simulink model "UseCase_v3"  (R2024b)
settings: Solver=ode1  StartTime=0.0  StopTime=365*24  FixedStep=0.05  RelTol=1e-3
libraries: filter_lib x5, buffer_lib x3, storage_lib x2, transport_lib x1
settings Model: SimulationMode=accelerator  Creator=marcv  LastModifiedBy=marcv
settings RTWCC: GPUComputeCapability=3.5

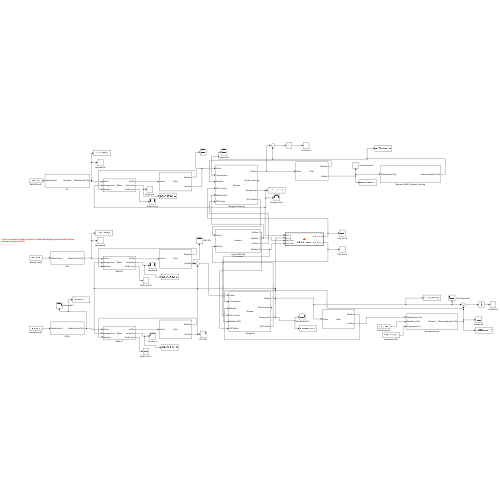
[thumbnail: Simulink's stored preview of the top-level diagram]
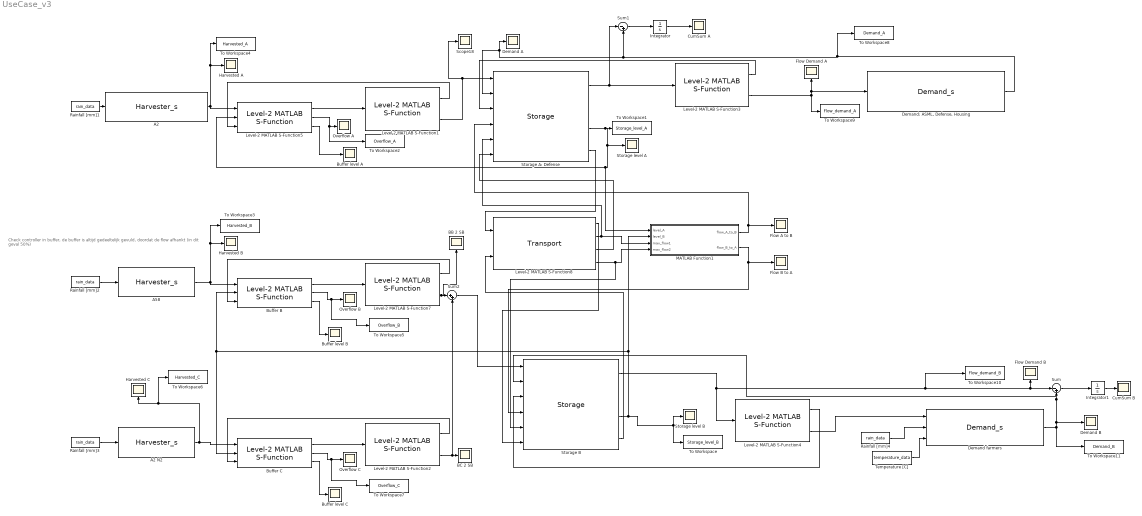
== system UseCase_v3 ==
  note: Check controller in buffer, de buffer is altijd gedeeltelijk gevuld, doordat de flow afhankt (in dit geval 50%)
  A2 : M-S-Function  FunctionName=Harvester_s  Parameters=Type_harvester, inflow_groundwater, Area  mask{Type_harvester=Dependant on ground water (tunnel), inflow_groundwater=91, Area=64000}
      mask prompts: Type_harvester "Type of harvester:"; inflow_groundwater "Inflow groundwater [m^3/h]:"; Area "Area [m^2]:"
      mask DialogControl DescGroupVar Prompt: Harvester
      mask DialogControl DescTextVar Prompt: Text
      mask Display:
      | disp('Harvester')
      | port_label('input', 1, 'Rainfall [mm]');
      | port_label('output', 1, 'Waterflow [m^3/h]');
  A2 N2 : M-S-Function  FunctionName=Harvester_s  Parameters=Type_harvester, inflow_groundwater, Area  mask{Type_harvester=Independant on ground water (resevoir, road ect.), inflow_groundwater=20, Area=21e4}
      mask prompts: Type_harvester "Type of harvester:"; inflow_groundwater "Inflow groundwater [m^3/h]:"; Area "Area [m^2]:"
      mask DialogControl DescGroupVar Prompt: Harvester
      mask DialogControl DescTextVar Prompt: Text
      mask Display:
      | port_label('input', 1, 'Rainfall [mm]');
      | port_label('output', 1, 'Waterflow [m^3/h]');
  A58 : M-S-Function  FunctionName=Harvester_s  Parameters=Type_harvester, inflow_groundwater, Area  mask{Type_harvester=Independant on ground water (resevoir, road ect.), inflow_groundwater=20, Area=13.5e4}
      mask prompts: Type_harvester "Type of harvester:"; inflow_groundwater "Inflow groundwater [m^3/h]:"; Area "Area [m^2]:"
      mask DialogControl DescGroupVar Prompt: Harvester
      mask DialogControl DescTextVar Prompt: Text
      mask Display:
      | port_label('input', 1, 'Rainfall [mm]');
      | port_label('output', 1, 'Waterflow [m^3/h]');
  BB 2 SB : Scope
  BC 2 SB : Scope
  Buffer B : buffer_lib/Level-2 MATLAB S-Function  Parameter1=7e3
  Buffer C : buffer_lib/Level-2 MATLAB S-Function  Parameter1=1e4
  Buffer level A : Scope
  Buffer level B : Scope
  Buffer level C : Scope
  CumSum A : Scope
  CumSum B : Scope
  Demand A : Scope
  Demand B : Scope
  Demand farmers : M-S-Function  FunctionName=Demand_s  Parameters=Type_demand, Constant_demand, Crop_type, Area  mask{Type_demand=Agriculture, Constant_demand=0, Crop_type=Potato, Area=3e5}
      mask prompts: Type_demand "Type of demand:"; Constant_demand "Demand [m^3/y]:"; Crop_type "Crop type:"; Area "Area [m^2]:"
      mask DialogControl DescGroupVar Prompt: Demand
      mask DialogControl DescTextVar Prompt: Demand text
      mask Display:
      | disp('Demand')
      | 
      | port_label('input', 1, 'Waterflow [m^3/h]');
      | if get_param(gcb, 'Type_demand') == "Agriculture"
      |     port_label('input', 2, 'Rainfall [m^3/h]');
      |     port_label('input', 3, 'Temperature [C]');
      | end
      | 
      | port_label('output', 1, 'Water demand [m^3/h]');
  "Demand: ASML, Defense, Housing" : M-S-Function  FunctionName=Demand_s  Parameters=Type_demand, Constant_demand, Crop_type, Area  mask{Type_demand=Constant demand, Constant_demand=8e5, Crop_type=Spinach, Area=3500000}
      mask prompts: Type_demand "Type of demand:"; Constant_demand "Demand [m^3/y]:"; Crop_type "Crop type:"; Area "Area [m^2]:"
      mask DialogControl DescGroupVar Prompt: Demand
      mask DialogControl DescTextVar Prompt: Demand text
      mask Display:
      | port_label('input', 1, 'Waterflow [m^3/h]');
      | if get_param(gcb, 'Type_demand') == "Agriculture"
      |     port_label('input', 2, 'Rainfall [m^3/h]');
      | end
      | 
      | port_label('output', 1, 'Water demand [m^3/h]');
  Flow A to B : Scope
  Flow B to A : Scope
  Flow Demand A : Scope
  Flow Demand B : Scope
  Harvested A : Scope
  Harvested B : Scope
  Harvested C : Scope
  Integrator : Integrator
  Integrator1 : Integrator
  Level-2 MATLAB S-Function1 : filter_lib/Level-2 MATLAB S-Function  filteroption=Custom filter  Parameter4=Cyclone-sand-UV [90 m3/h]  Parameter1=200  Parameter2=1
  Level-2 MATLAB S-Function2 : filter_lib/Level-2 MATLAB S-Function  filteroption=Custom filter  Parameter4=Cyclone-sand-UV [90 m3/h]  Parameter1=100  Parameter2=1
  Level-2 MATLAB S-Function3 : filter_lib/Level-2 MATLAB S-Function  filteroption=Custom filter  Parameter4=Cyclone-sand-UV [90 m3/h]  Parameter1=100  Parameter2=1
  Level-2 MATLAB S-Function4 : filter_lib/Level-2 MATLAB S-Function  filteroption=Custom filter  Parameter4=Cyclone-sand-UV [90 m3/h]  Parameter1=400  Parameter2=1
  Level-2 MATLAB S-Function5 : buffer_lib/Level-2 MATLAB S-Function  Parameter1=1e4
  Level-2 MATLAB S-Function7 : filter_lib/Level-2 MATLAB S-Function  filteroption=Custom filter  Parameter4=Cyclone-sand-UV [90 m3/h]  Parameter1=100  Parameter2=1
  Level-2 MATLAB S-Function8 : transport_lib/Transport  max_flow_result1=195.5517  max_flow_result2=188.5717  flowDirec=Bidirectional  setupopt=Transport only  Transporttype=Custom  Dist=20000  elevation=1  width=1  depth=3  diameter=0.3  dP=3  customflow=200  filteroption=Common filter  Fflowmax=3000  dPfilter=1  selectedfilter=Reverse Osmosis [27 m3/h (PureAqua TW-173K-4680)]  filterparallel=2
  MATLAB Function1 : MATLAB Function  TreatAsAtomicUnit=on
  Overflow A : Scope
  Overflow B : Scope
  Overflow C : Scope
  Rainfall [mm]{1..4} (4 alike) : FromWorkspace  VariableName=rain_data  OutDataTypeStr=double  SampleTime=1
  Scope18 : Scope
  Storage A: Defense : storage_lib/Storage  Parameter1=22.5e4  Parameter2=0.6  Parameter3=1 interconnection
  Storage B : storage_lib/Storage  Parameter1=5e4  Parameter2=0.6  Parameter3=1 interconnection
  Storage level A : Scope
  Storage level B : Scope
  Sum : Sum  Inputs=|-+
  Sum1 : Sum  Inputs=|-+
  Sum2 : Sum  Inputs=|++
  Temperature [C] : FromWorkspace  VariableName=temperature_data  OutDataTypeStr=double  SampleTime=1
  To Workspace : ToWorkspace  VariableName=Storage_level_B  SampleTime=1
  To Workspace1 : ToWorkspace  VariableName=Storage_level_A  SampleTime=1
  To Workspace10 : ToWorkspace  VariableName=Flow_demand_B  SampleTime=1
  To Workspace11 : ToWorkspace  VariableName=Demand_B  SampleTime=1
  To Workspace2 : ToWorkspace  VariableName=Overflow_A  SampleTime=1
  To Workspace3 : ToWorkspace  VariableName=Harvested_B  SampleTime=1
  To Workspace4 : ToWorkspace  VariableName=Harvested_A  SampleTime=1
  To Workspace5 : ToWorkspace  VariableName=Overflow_B  SampleTime=1
  To Workspace6 : ToWorkspace  VariableName=Harvested_C  SampleTime=1
  To Workspace7 : ToWorkspace  VariableName=Overflow_C  SampleTime=1
  To Workspace8 : ToWorkspace  VariableName=Demand_A  SampleTime=1
  To Workspace9 : ToWorkspace  VariableName=Flow_demand_A  SampleTime=1
  wires:
  Rainfall [mm]1/1 -> A2/1
  A2/1 -> To Workspace4/1, Harvested A/1, Level-2 MATLAB S-Function5/1
  Level-2 MATLAB S-Function5/3 -> Buffer level A/1
  Level-2 MATLAB S-Function1/1 -> Level-2 MATLAB S-Function5/3
  Level-2 MATLAB S-Function5/1 -> Level-2 MATLAB S-Function1/1
  Level-2 MATLAB S-Function5/2 -> To Workspace2/1, Overflow A/1
  Level-2 MATLAB S-Function1/2 -> Storage A: Defense/1, Scope18/1
  Storage A: Defense/1 -> Level-2 MATLAB S-Function3/1, Sum1/1
  Storage A: Defense/3 -> To Workspace1/1, MATLAB Function1/1(level_A), Level-2 MATLAB S-Function5/2, Storage level A/1
  Storage B/3 -> To Workspace/1, Storage level B/1, MATLAB Function1/2(level_B), Buffer B/2, Buffer C/2
  Buffer B/2 -> To Workspace5/1, Overflow B/1
  Buffer B/1 -> Level-2 MATLAB S-Function7/1
  Level-2 MATLAB S-Function7/1 -> Buffer B/3
  A58/1 -> To Workspace3/1, Harvested B/1, Buffer B/1
  Buffer B/3 -> Buffer level B/1
  Rainfall [mm]2/1 -> A58/1
  "Demand: ASML, Defense, Housing"/1 -> Demand A/1, Storage A: Defense/2, Sum1/2, To Workspace8/1
  Demand farmers/1 -> Storage B/2, Sum/2, Demand B/1, To Workspace11/1
  Storage B/1 -> To Workspace10/1, Sum/1, Flow Demand B/1, Level-2 MATLAB S-Function4/1
  Rainfall [mm]4/1 -> Demand farmers/2
  Sum1/1 -> Integrator/1
  Integrator/1 -> CumSum A/1
  Integrator1/1 -> CumSum B/1
  Sum/1 -> Integrator1/1
  Level-2 MATLAB S-Function2/1 -> Buffer C/3
  Buffer C/2 -> To Workspace7/1, Overflow C/1
  Rainfall [mm]3/1 -> A2 N2/1
  Buffer C/1 -> Level-2 MATLAB S-Function2/1
  Buffer C/3 -> Buffer level C/1
  A2 N2/1 -> Buffer C/1, To Workspace6/1, Harvested C/1
  Level-2 MATLAB S-Function7/2 -> BB 2 SB/1, Sum2/1
  Sum2/1 -> Storage B/1
  Level-2 MATLAB S-Function2/2 -> BC 2 SB/1, Sum2/2
  Temperature [C]/1 -> Demand farmers/3
  Level-2 MATLAB S-Function3/1 -> Storage A: Defense/3
  Level-2 MATLAB S-Function3/2 -> To Workspace9/1, "Demand: ASML, Defense, Housing"/1, Flow Demand A/1
  Level-2 MATLAB S-Function4/2 -> Demand farmers/1
  Level-2 MATLAB S-Function4/1 -> Storage B/3
  Level-2 MATLAB S-Function8/2 -> Storage A: Defense/5, MATLAB Function1/3(max_flow1)
  Level-2 MATLAB S-Function8/4 -> Storage B/5, MATLAB Function1/4(max_flow2)
  MATLAB Function1/1(flow_A_to_B) -> Storage A: Defense/4, Flow A to B/1
  Storage A: Defense/4 -> Level-2 MATLAB S-Function8/1
  Level-2 MATLAB S-Function8/1 -> Storage B/6
  MATLAB Function1/2(flow_B_to_A) -> Flow B to A/1, Storage B/4
  Storage B/4 -> Level-2 MATLAB S-Function8/2
  Level-2 MATLAB S-Function8/3 -> Storage A: Defense/6

== matlab function UseCase_v3/MATLAB Function1 ==
  data: level_A input; flow_A_to_B output; level_B input; max_flow1 input; max_flow2 input; flow_B_to_A output
function [flow_A_to_B, flow_B_to_A] = real_time_control(level_A, level_B, max_flow1, max_flow2)

thresholdA = 0.05;
thresholdB = 0.05;

% min_threshold = 0;
flow_A_to_B = 0;
flow_B_to_A = 0;
gain = 3;

% Flow from A to B
if (level_A > level_B) && (level_A > thresholdA)
    flow_A_to_B = min(gain*(level_A - level_B), 1) * max_flow1;


% Flow from B to A
elseif (level_B > level_A) && (level_B > thresholdB)
    flow_B_to_A = min(gain*(level_B - level_A), 1) * max_flow2;

% elseif (level_A > level_B) && (level_B < min_threshold)
%     flow_A_to_B = min((level_A - level_B), 1) * max_flow1;
% 
% elseif (level_B > level_A) && (level_A < min_threshold)
%     flow_B_to_A = min((level_B - level_A), 1) * max_flow2;


end
